simulink model "FlFWLvl_DD"  (R2016b)
settings: configuration reference "CodeGenConfigSet" (kept outside this file)
values from neighbouring files (symbols this model uses):
  FlFWLvl_tiSensSigRawDebHiLo_C = Calibration.Parameter    [init_FlFWLvl_DD.m]    (also in init_FlFWLvl_DD_SIL.m = Simulink.Parameter)
  FlFWLvl_tiSensSigRawDebLoHi_C = Calibration.Parameter    [init_FlFWLvl_DD.m]    (also in init_FlFWLvl_DD_SIL.m = Simulink.Parameter)
undefined symbols (not defined in the file or in its folder): FlFWLvl_DD_DT
libraries: CXLib x1
settings Model: Creator=胡炎林  LastModifiedBy=liutao
settings ConfigSetRef: SourceLocation=Base Workspace

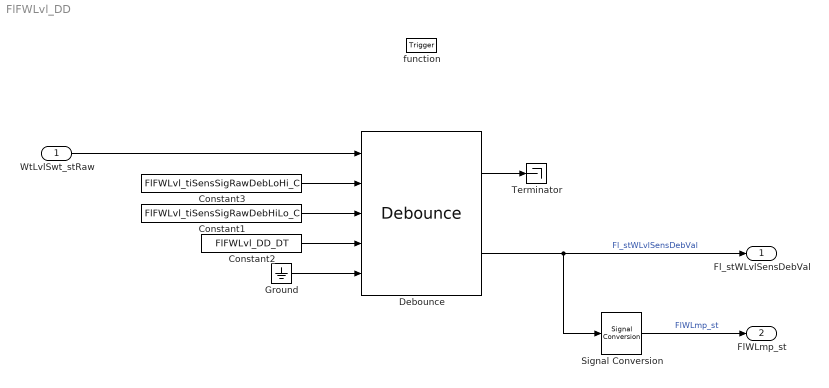
== system FlFWLvl_DD ==
  WtLvlSwt_stRaw : Inport  Description=CAN interface message for the status of water in fuel  OutMin=0  OutMax=1  OutDataTypeStr=boolean
  function : TriggerPort  TriggerType=function-call  VariantControl=Variant
  Constant1 : Constant  Value=FlFWLvl_tiSensSigRawDebHiLo_C
  Constant2 : Constant  Value=FlFWLvl_DD_DT
  Constant3 : Constant  Value=FlFWLvl_tiSensSigRawDebLoHi_C
  Debounce : CXLib/Debounce
  Ground : Ground
  Signal Conversion : SignalConversion  OverrideOpt=off
  Terminator : Terminator
  Fl_stWLvlSensDebVal : Outport  Description=Debounced value of fuel filter water level sensor signal  OutMin=0  OutMax=1  OutDataTypeStr=boolean
  FlWLmp_st : Outport  Description=Status of Water Level Indication lamp  Port=2  OutMin=0  OutMax=1  OutDataTypeStr=boolean
  wires:
  WtLvlSwt_stRaw/1 -> Debounce/1
  Constant3/1 -> Debounce/2
  Constant1/1 -> Debounce/3
  Constant2/1 -> Debounce/4
  Ground/1 -> Debounce/5
  Debounce/1 -> Terminator/1
  Debounce/2 -> Signal Conversion/1, Fl_stWLvlSensDebVal/1  "Fl_stWLvlSensDebVal"
  Signal Conversion/1 -> FlWLmp_st/1  "FlWLmp_st"
